simulink model "sim_battery_pack_simulink_with_EV_Load"  (R2021b)
settings: Solver=FixedStepAuto  StartTime=0.0  StopTime=3460.480  FixedStep=0.01  RelTol=1e-3
values from neighbouring files (symbols this model uses):
  Af = 1.4*1.6    (= 2.24)    [battery_pack_init_18_11.m]
  b = 0.002    [battery_pack_init_18_11.m]
  Batt_Eff = .98    (= 0.98)    [battery_pack_init_18_11.m]
  Batt_Ene_Cap = 7.37    [battery_pack_init_18_11.m]
  cd = 0.45    [battery_pack_init_18_11.m]
  dt = 0.01    [battery_pack_init_18_11.m]
  g = 9.81    [battery_pack_init_18_11.m]
  Gr = 5.75*.85    (= 4.8875)    [battery_pack_init_18_11.m]
  Grade = 7    [battery_pack_init_18_11.m]
  Ini_SOC = 100    [battery_pack_init_18_11.m]
  kappa = 0.1    [battery_pack_init_18_11.m]
  M = M_k+M_P    (= 445)    [battery_pack_init_18_11.m]
  M_Trq = T_m    [battery_pack_init_18_11.m]
  M_w = w_m    [battery_pack_init_18_11.m]
  Mot_Eff = .9    (= 0.9)    [battery_pack_init_18_11.m]
  mu = 0.016    [battery_pack_init_18_11.m]
  Np = 7    [battery_pack_init_18_11.m]
  Ns = 12    [battery_pack_init_18_11.m]
  Qgain = 1    [battery_pack_init_18_11.m]
  R0 = zeros(numpoles,1)    [battery_pack_init_18_11.m]
  R0Param = getParamESC('R0Param',T,cell_model)    [battery_pack_init_18_11.m]
  R_w = .3048/2    (= 0.1524)    [battery_pack_init_18_11.m]
  Re_spe_max = 50*5/18    (= 13.8888888889)    [battery_pack_init_18_11.m]
  Re_spe_min = 0*5/18    (= 0)    [battery_pack_init_18_11.m]
  rho = 1.225    [battery_pack_init_18_11.m]
  rt = .0008    (= 0.0008)    [battery_pack_init_18_11.m]
  T = 40    [battery_pack_init_18_11.m]
  T_MIDC = T_MIDC(1:72)    [battery_pack_init_18_11.m]
  Trans_Eff = .95    (= 0.95)    [battery_pack_init_18_11.m]
  V_MIDC = V_MIDC(1:72)    [battery_pack_init_18_11.m]
  Z0 = 0.75 + (1-0.75).*rand(1,Np)    [battery_pack_init_18_11.m]
undefined symbols (not defined in the file or in its folder): cell_model, FLbattery, gain, iload, sigbuilder_block, VMIDC
libraries: simulink x16, autolibshared x2, slpidlib x1, simulink_extras x1
(part 12 of 17)

== matlab function sim_battery_pack_simulink_with_EV_Load/SCM6/cell10/cell_model ==
  data: vk output size=1; T input; deltaT input; iR0 input; zkp input; irkp input; irkc output size=3; zkc output size=1; OCV output size=1; cell_model parameter; ik input; Qgain parameter

% function [vk,irk,hk,zk,sik,OCV] = simCell(ik,T,deltaT,model,z0,iR0,h0)
% 
% Simulates an ESC model for input current ik at temperature T
%
% Inputs:  ik - current, where (+) is discharge
%          T  - temperature (degC)
%      deltaT - sampling interval in data (s)
%       model - standard model structure
%          z0 - initial cell state of charge
%         iR0 - initial resistor currents as column vector
%          h0 - initial hysteresis state
% Outputs: vk - cell voltage for all timesteps
%         irk - resistor currents (in R-C branches) for all timesteps
%          hk - hysteresis states for all timesteps
%          zk - state of charge for all timesteps
%         sik - instantaneous hysteresis for all timesteps
%         OCV - open-circuit voltage for all timesteps

% Copyright (c) 2015 by Gregory L. Plett of the University of Colorado 
% Colorado Springs (UCCS). This work is licensed under a Creative Commons 
% Attribution-NonCommercial-ShareAlike 4.0 Intl. License, v. 1.0.
% It is provided "as is", without express or implied warranty, for 
% educational and informational purposes only.
%
% This file is provided as a supplement to: Plett, Gregory L., "Battery
% Management Systems, Volume I, Battery Modeling," Artech House, 2015.

function [vk,irkc,zkc,OCV] = cellmodel(T,deltaT,iR0, zkp,irkp, cell_model,ik, Qgain)
  % Force data to be column vector(s)
  
%   ik=[DYNData.script1.current(round(t*10)),DYNData.script1.current(round(t*10)+1)];
%   ik=interp1(0.1*(1:length(DYNData.script1.current)),DYNData.script1.current,t,'nearest');
  ik = ik(:); iR0 = iR0(:);
  
  % Get model parameters from model structure
  RCfact = exp(-deltaT./abs(getParamESC('RCParam',T,cell_model)))';
  Q = Qgain* getParamESC('QParam',T,cell_model);
  RParam = getParamESC('RParam',T,cell_model);
  R0Param = getParamESC('R0Param',T,cell_model);
  etaParam = getParamESC('etaParam',T,cell_model);
  
  etaik = ik; 
  for iii=1:length(ik)
    if etaik(iii)<0
        etaik(iii) = etaParam*ik(iii); % compensate for coulombic efficiency
    end
  end
  % Simulate the dynamic states of the model
  %if exist('ss','file'), % use control-system-toolbox method, if available
%     sysd= ss(diag(RCfact),1-RCfact,eye(length(RCfact)),0,0.1);
%     irk = lsim(sysd,etaik,[],iR0);
  %else
    irkc = RCfact.*irkp + (1-RCfact)*etaik(1);
  %end
%    irkc2 = irk(2,:)';
%    irkc=(irkc1+irkc2)/2;
  zkc = zkp-etaik(1)*deltaT/(Q*3600); 

    
  % Compute output equation
  OCV = OCVfromSOCtemp(zkc,T,cell_model);
  vk = OCV - RParam*irkc - ik(1).*R0Param ;%+ M*hk + M0*sik;
  
  


function theParam = getParamESC(paramName,temp,model)
%   theFields = fields(model); % get list of fields stored in model
%   match = strcmpi(paramName,theFields); % see if any match desired data
%   if ~match, % if not, throw an error
%     error('Parameter "%s" does not exist in model',paramName);
%   end
%   fieldName = char(theFields(match)); % case-sensitive field name

  % if model contains data at only one temperature
  if isscalar(model.temps),
    if model.temps ~= temp, % check whether requested data exists
      error('Model does not contain requested data at this temperature');
    end
    theParam = model.(paramName);
    return
  end

  % Otherwise, model has multiple temperatures. Bound input "temp" between
  % mininum and maximum stored temperature to prohibit "NaN" in output
  theParamData = model.(paramName);
  temp = max(min(temp,max(model.temps)),min(model.temps)); 
  ind = find(model.temps == temp); % see if there is an exact match to
  if ~isempty(ind), % avoid call to (slow) interp1 whenever possible
    if size(theParamData,1) == 1,
      theParam = theParamData(ind);
    else
      theParam = theParamData(ind,:);
    end
  else % if there is not an exact match, we interpolate between parameter
    theParam = interp1(model.temps,theParamData,temp,'spline'); % values
  end  % stored at different temperatures
  
  % function ocv = OCVfromSOCtemp(soc,temp,model)
%
% Computes the fully rested open-circuit voltage for a particular state of 
% charge and temperature point
%
% Inputs: soc = scalar or matrix of cell state of charge points
%        temp = scalar or matrix of temperatures at which to calc. OCV
%       model = data structure produced by processDynamic
% Output: ocv = scalar or matrix of open circuit voltages -- one for every
%               soc and temperature input point

% Copyright (c) 2015 by Gregory L. Plett of the University of Colorado 
% Colorado Springs (UCCS). This work is licensed under a Creative Commons 
% Attribution-NonCommercial-ShareAlike 4.0 Intl. License, v. 1.0.
% It is provided "as is", without express or implied warranty, for 
% educational and informational purposes only.
%
% This file is provided as a supplement to: Plett, Gregory L., "Battery
% Management Systems, Volume I, Battery Modeling," Artech House, 2015.

function ocv=OCVfromSOCtemp(soc,temp,model)
  soccol = soc(:); % force soc to be column vector
  SOC = model.SOC(:); % force to be column vector
  OCV0 = model.OCV0(:); % force to be column vector
  OCVrel = model.OCVrel(:); % force to be column vector
  if isscalar(temp), % replicate a scalar temperature for all socs
    tempcol = temp*ones(size(soccol)); 
  else
    tempcol = temp(:); % force matrix temperature to be column vector
    if ~isequal(size(tempcol),size(soccol)),
      error(['Function inputs "soc" and "temp" must either have same '...
        'number of elements, or "temp" must be a scalar']);
    end
  end
  diffSOC=SOC(2)-SOC(1); % spacing between SOC points - assume uniform
  ocv=zeros(size(soccol)); % initialize output to zero
  I1=find(soccol <= SOC(1)); % indices of socs below model-stored data
  I2=find(soccol >= SOC(end)); % and of socs above model-stored data
  I3=find(soccol > SOC(1) & soccol < SOC(end)); % the rest of them
  I6=isnan(soccol); % if input is "not a number" for any locations

  % for voltages less than lowest stored soc datapoint, extrapolate off 
  % low end of table 
  if ~isempty(I1),
    dv = (OCV0(2)+tempcol.*OCVrel(2)) - (OCV0(1)+tempcol.*OCVrel(1));
    ocv(I1)= (soccol(I1)-SOC(1)).*dv(I1)/diffSOC + ...
             OCV0(1)+tempcol(I1).*OCVrel(1);
  end

  % for voltages greater than highest stored soc datapoint, extrapolate off
  % high end of table
  if ~isempty(I2),
    dv = (OCV0(end)+tempcol.*OCVrel(end)) - ...
         (OCV0(end-1)+tempcol.*OCVrel(end-1));
    ocv(I2) = (soccol(I2)-SOC(end)).*dv(I2)/diffSOC + ...
              OCV0(end)+tempcol(I2).*OCVrel(end);
  end

  % for normal soc range, manually interpolate (10x faster than "interp1")
  I4=(soccol(I3)-SOC(1))/diffSOC; % using linear interpolation
  I5=floor(I4); I45 = I4-I5; omI45 = 1-I45;
  ocv(I3)=OCV0(I5+1).*omI45 + OCV0(I5+2).*I45;
  ocv(I3)=ocv(I3) + tempcol(I3).*(OCVrel(I5+1).*omI45 + OCVrel(I5+2).*I45);
  ocv(I6)=0; % replace NaN SOCs with zero voltage
  ocv = reshape(ocv,size(soc)); % output is same shape as input

== matlab function sim_battery_pack_simulink_with_EV_Load/SCM6/cell11/cell_model ==
  data: vk output size=1; T input; deltaT input; iR0 input; zkp input; irkp input; irkc output size=3; zkc output size=1; OCV output size=1; cell_model parameter; ik input; Qgain parameter

% function [vk,irk,hk,zk,sik,OCV] = simCell(ik,T,deltaT,model,z0,iR0,h0)
% 
% Simulates an ESC model for input current ik at temperature T
%
% Inputs:  ik - current, where (+) is discharge
%          T  - temperature (degC)
%      deltaT - sampling interval in data (s)
%       model - standard model structure
%          z0 - initial cell state of charge
%         iR0 - initial resistor currents as column vector
%          h0 - initial hysteresis state
% Outputs: vk - cell voltage for all timesteps
%         irk - resistor currents (in R-C branches) for all timesteps
%          hk - hysteresis states for all timesteps
%          zk - state of charge for all timesteps
%         sik - instantaneous hysteresis for all timesteps
%         OCV - open-circuit voltage for all timesteps

% Copyright (c) 2015 by Gregory L. Plett of the University of Colorado 
% Colorado Springs (UCCS). This work is licensed under a Creative Commons 
% Attribution-NonCommercial-ShareAlike 4.0 Intl. License, v. 1.0.
% It is provided "as is", without express or implied warranty, for 
% educational and informational purposes only.
%
% This file is provided as a supplement to: Plett, Gregory L., "Battery
% Management Systems, Volume I, Battery Modeling," Artech House, 2015.

function [vk,irkc,zkc,OCV] = cellmodel(T,deltaT,iR0, zkp,irkp, cell_model,ik, Qgain)
  % Force data to be column vector(s)
  
%   ik=[DYNData.script1.current(round(t*10)),DYNData.script1.current(round(t*10)+1)];
%   ik=interp1(0.1*(1:length(DYNData.script1.current)),DYNData.script1.current,t,'nearest');
  ik = ik(:); iR0 = iR0(:);
  
  % Get model parameters from model structure
  RCfact = exp(-deltaT./abs(getParamESC('RCParam',T,cell_model)))';
  Q = Qgain* getParamESC('QParam',T,cell_model);
  RParam = getParamESC('RParam',T,cell_model);
  R0Param = getParamESC('R0Param',T,cell_model);
  etaParam = getParamESC('etaParam',T,cell_model);
  
  etaik = ik; 
  for iii=1:length(ik)
    if etaik(iii)<0
        etaik(iii) = etaParam*ik(iii); % compensate for coulombic efficiency
    end
  end
  % Simulate the dynamic states of the model
  %if exist('ss','file'), % use control-system-toolbox method, if available
%     sysd= ss(diag(RCfact),1-RCfact,eye(length(RCfact)),0,0.1);
%     irk = lsim(sysd,etaik,[],iR0);
  %else
    irkc = RCfact.*irkp + (1-RCfact)*etaik(1);
  %end
%    irkc2 = irk(2,:)';
%    irkc=(irkc1+irkc2)/2;
  zkc = zkp-etaik(1)*deltaT/(Q*3600); 

    
  % Compute output equation
  OCV = OCVfromSOCtemp(zkc,T,cell_model);
  vk = OCV - RParam*irkc - ik(1).*R0Param ;%+ M*hk + M0*sik;
  
  


function theParam = getParamESC(paramName,temp,model)
%   theFields = fields(model); % get list of fields stored in model
%   match = strcmpi(paramName,theFields); % see if any match desired data
%   if ~match, % if not, throw an error
%     error('Parameter "%s" does not exist in model',paramName);
%   end
%   fieldName = char(theFields(match)); % case-sensitive field name

  % if model contains data at only one temperature
  if isscalar(model.temps),
    if model.temps ~= temp, % check whether requested data exists
      error('Model does not contain requested data at this temperature');
    end
    theParam = model.(paramName);
    return
  end

  % Otherwise, model has multiple temperatures. Bound input "temp" between
  % mininum and maximum stored temperature to prohibit "NaN" in output
  theParamData = model.(paramName);
  temp = max(min(temp,max(model.temps)),min(model.temps)); 
  ind = find(model.temps == temp); % see if there is an exact match to
  if ~isempty(ind), % avoid call to (slow) interp1 whenever possible
    if size(theParamData,1) == 1,
      theParam = theParamData(ind);
    else
      theParam = theParamData(ind,:);
    end
  else % if there is not an exact match, we interpolate between parameter
    theParam = interp1(model.temps,theParamData,temp,'spline'); % values
  end  % stored at different temperatures
  
  % function ocv = OCVfromSOCtemp(soc,temp,model)
%
% Computes the fully rested open-circuit voltage for a particular state of 
% charge and temperature point
%
% Inputs: soc = scalar or matrix of cell state of charge points
%        temp = scalar or matrix of temperatures at which to calc. OCV
%       model = data structure produced by processDynamic
% Output: ocv = scalar or matrix of open circuit voltages -- one for every
%               soc and temperature input point

% Copyright (c) 2015 by Gregory L. Plett of the University of Colorado 
% Colorado Springs (UCCS). This work is licensed under a Creative Commons 
% Attribution-NonCommercial-ShareAlike 4.0 Intl. License, v. 1.0.
% It is provided "as is", without express or implied warranty, for 
% educational and informational purposes only.
%
% This file is provided as a supplement to: Plett, Gregory L., "Battery
% Management Systems, Volume I, Battery Modeling," Artech House, 2015.

function ocv=OCVfromSOCtemp(soc,temp,model)
  soccol = soc(:); % force soc to be column vector
  SOC = model.SOC(:); % force to be column vector
  OCV0 = model.OCV0(:); % force to be column vector
  OCVrel = model.OCVrel(:); % force to be column vector
  if isscalar(temp), % replicate a scalar temperature for all socs
    tempcol = temp*ones(size(soccol)); 
  else
    tempcol = temp(:); % force matrix temperature to be column vector
    if ~isequal(size(tempcol),size(soccol)),
      error(['Function inputs "soc" and "temp" must either have same '...
        'number of elements, or "temp" must be a scalar']);
    end
  end
  diffSOC=SOC(2)-SOC(1); % spacing between SOC points - assume uniform
  ocv=zeros(size(soccol)); % initialize output to zero
  I1=find(soccol <= SOC(1)); % indices of socs below model-stored data
  I2=find(soccol >= SOC(end)); % and of socs above model-stored data
  I3=find(soccol > SOC(1) & soccol < SOC(end)); % the rest of them
  I6=isnan(soccol); % if input is "not a number" for any locations

  % for voltages less than lowest stored soc datapoint, extrapolate off 
  % low end of table 
  if ~isempty(I1),
    dv = (OCV0(2)+tempcol.*OCVrel(2)) - (OCV0(1)+tempcol.*OCVrel(1));
    ocv(I1)= (soccol(I1)-SOC(1)).*dv(I1)/diffSOC + ...
             OCV0(1)+tempcol(I1).*OCVrel(1);
  end

  % for voltages greater than highest stored soc datapoint, extrapolate off
  % high end of table
  if ~isempty(I2),
    dv = (OCV0(end)+tempcol.*OCVrel(end)) - ...
         (OCV0(end-1)+tempcol.*OCVrel(end-1));
    ocv(I2) = (soccol(I2)-SOC(end)).*dv(I2)/diffSOC + ...
              OCV0(end)+tempcol(I2).*OCVrel(end);
  end

  % for normal soc range, manually interpolate (10x faster than "interp1")
  I4=(soccol(I3)-SOC(1))/diffSOC; % using linear interpolation
  I5=floor(I4); I45 = I4-I5; omI45 = 1-I45;
  ocv(I3)=OCV0(I5+1).*omI45 + OCV0(I5+2).*I45;
  ocv(I3)=ocv(I3) + tempcol(I3).*(OCVrel(I5+1).*omI45 + OCVrel(I5+2).*I45);
  ocv(I6)=0; % replace NaN SOCs with zero voltage
  ocv = reshape(ocv,size(soc)); % output is same shape as input

== matlab function sim_battery_pack_simulink_with_EV_Load/SCM6/cell12/cell_model ==
  data: vk output size=1; T input; deltaT input; iR0 input; zkp input; irkp input; irkc output size=3; zkc output size=1; OCV output size=1; cell_model parameter; ik input; Qgain parameter

% function [vk,irk,hk,zk,sik,OCV] = simCell(ik,T,deltaT,model,z0,iR0,h0)
% 
% Simulates an ESC model for input current ik at temperature T
%
% Inputs:  ik - current, where (+) is discharge
%          T  - temperature (degC)
%      deltaT - sampling interval in data (s)
%       model - standard model structure
%          z0 - initial cell state of charge
%         iR0 - initial resistor currents as column vector
%          h0 - initial hysteresis state
% Outputs: vk - cell voltage for all timesteps
%         irk - resistor currents (in R-C branches) for all timesteps
%          hk - hysteresis states for all timesteps
%          zk - state of charge for all timesteps
%         sik - instantaneous hysteresis for all timesteps
%         OCV - open-circuit voltage for all timesteps

% Copyright (c) 2015 by Gregory L. Plett of the University of Colorado 
% Colorado Springs (UCCS). This work is licensed under a Creative Commons 
% Attribution-NonCommercial-ShareAlike 4.0 Intl. License, v. 1.0.
% It is provided "as is", without express or implied warranty, for 
% educational and informational purposes only.
%
% This file is provided as a supplement to: Plett, Gregory L., "Battery
% Management Systems, Volume I, Battery Modeling," Artech House, 2015.

function [vk,irkc,zkc,OCV] = cellmodel(T,deltaT,iR0, zkp,irkp, cell_model,ik, Qgain)
  % Force data to be column vector(s)
  
%   ik=[DYNData.script1.current(round(t*10)),DYNData.script1.current(round(t*10)+1)];
%   ik=interp1(0.1*(1:length(DYNData.script1.current)),DYNData.script1.current,t,'nearest');
  ik = ik(:); iR0 = iR0(:);
  
  % Get model parameters from model structure
  RCfact = exp(-deltaT./abs(getParamESC('RCParam',T,cell_model)))';
  Q = Qgain* getParamESC('QParam',T,cell_model);
  RParam = getParamESC('RParam',T,cell_model);
  R0Param = getParamESC('R0Param',T,cell_model);
  etaParam = getParamESC('etaParam',T,cell_model);
  
  etaik = ik; 
  for iii=1:length(ik)
    if etaik(iii)<0
        etaik(iii) = etaParam*ik(iii); % compensate for coulombic efficiency
    end
  end
  % Simulate the dynamic states of the model
  %if exist('ss','file'), % use control-system-toolbox method, if available
%     sysd= ss(diag(RCfact),1-RCfact,eye(length(RCfact)),0,0.1);
%     irk = lsim(sysd,etaik,[],iR0);
  %else
    irkc = RCfact.*irkp + (1-RCfact)*etaik(1);
  %end
%    irkc2 = irk(2,:)';
%    irkc=(irkc1+irkc2)/2;
  zkc = zkp-etaik(1)*deltaT/(Q*3600); 

    
  % Compute output equation
  OCV = OCVfromSOCtemp(zkc,T,cell_model);
  vk = OCV - RParam*irkc - ik(1).*R0Param ;%+ M*hk + M0*sik;
  
  


function theParam = getParamESC(paramName,temp,model)
%   theFields = fields(model); % get list of fields stored in model
%   match = strcmpi(paramName,theFields); % see if any match desired data
%   if ~match, % if not, throw an error
%     error('Parameter "%s" does not exist in model',paramName);
%   end
%   fieldName = char(theFields(match)); % case-sensitive field name

  % if model contains data at only one temperature
  if isscalar(model.temps),
    if model.temps ~= temp, % check whether requested data exists
      error('Model does not contain requested data at this temperature');
    end
    theParam = model.(paramName);
    return
  end

  % Otherwise, model has multiple temperatures. Bound input "temp" between
  % mininum and maximum stored temperature to prohibit "NaN" in output
  theParamData = model.(paramName);
  temp = max(min(temp,max(model.temps)),min(model.temps)); 
  ind = find(model.temps == temp); % see if there is an exact match to
  if ~isempty(ind), % avoid call to (slow) interp1 whenever possible
    if size(theParamData,1) == 1,
      theParam = theParamData(ind);
    else
      theParam = theParamData(ind,:);
    end
  else % if there is not an exact match, we interpolate between parameter
    theParam = interp1(model.temps,theParamData,temp,'spline'); % values
  end  % stored at different temperatures
  
  % function ocv = OCVfromSOCtemp(soc,temp,model)
%
% Computes the fully rested open-circuit voltage for a particular state of 
% charge and temperature point
%
% Inputs: soc = scalar or matrix of cell state of charge points
%        temp = scalar or matrix of temperatures at which to calc. OCV
%       model = data structure produced by processDynamic
% Output: ocv = scalar or matrix of open circuit voltages -- one for every
%               soc and temperature input point

% Copyright (c) 2015 by Gregory L. Plett of the University of Colorado 
% Colorado Springs (UCCS). This work is licensed under a Creative Commons 
% Attribution-NonCommercial-ShareAlike 4.0 Intl. License, v. 1.0.
% It is provided "as is", without express or implied warranty, for 
% educational and informational purposes only.
%
% This file is provided as a supplement to: Plett, Gregory L., "Battery
% Management Systems, Volume I, Battery Modeling," Artech House, 2015.

function ocv=OCVfromSOCtemp(soc,temp,model)
  soccol = soc(:); % force soc to be column vector
  SOC = model.SOC(:); % force to be column vector
  OCV0 = model.OCV0(:); % force to be column vector
  OCVrel = model.OCVrel(:); % force to be column vector
  if isscalar(temp), % replicate a scalar temperature for all socs
    tempcol = temp*ones(size(soccol)); 
  else
    tempcol = temp(:); % force matrix temperature to be column vector
    if ~isequal(size(tempcol),size(soccol)),
      error(['Function inputs "soc" and "temp" must either have same '...
        'number of elements, or "temp" must be a scalar']);
    end
  end
  diffSOC=SOC(2)-SOC(1); % spacing between SOC points - assume uniform
  ocv=zeros(size(soccol)); % initialize output to zero
  I1=find(soccol <= SOC(1)); % indices of socs below model-stored data
  I2=find(soccol >= SOC(end)); % and of socs above model-stored data
  I3=find(soccol > SOC(1) & soccol < SOC(end)); % the rest of them
  I6=isnan(soccol); % if input is "not a number" for any locations

  % for voltages less than lowest stored soc datapoint, extrapolate off 
  % low end of table 
  if ~isempty(I1),
    dv = (OCV0(2)+tempcol.*OCVrel(2)) - (OCV0(1)+tempcol.*OCVrel(1));
    ocv(I1)= (soccol(I1)-SOC(1)).*dv(I1)/diffSOC + ...
             OCV0(1)+tempcol(I1).*OCVrel(1);
  end

  % for voltages greater than highest stored soc datapoint, extrapolate off
  % high end of table
  if ~isempty(I2),
    dv = (OCV0(end)+tempcol.*OCVrel(end)) - ...
         (OCV0(end-1)+tempcol.*OCVrel(end-1));
    ocv(I2) = (soccol(I2)-SOC(end)).*dv(I2)/diffSOC + ...
              OCV0(end)+tempcol(I2).*OCVrel(end);
  end

  % for normal soc range, manually interpolate (10x faster than "interp1")
  I4=(soccol(I3)-SOC(1))/diffSOC; % using linear interpolation
  I5=floor(I4); I45 = I4-I5; omI45 = 1-I45;
  ocv(I3)=OCV0(I5+1).*omI45 + OCV0(I5+2).*I45;
  ocv(I3)=ocv(I3) + tempcol(I3).*(OCVrel(I5+1).*omI45 + OCVrel(I5+2).*I45);
  ocv(I6)=0; % replace NaN SOCs with zero voltage
  ocv = reshape(ocv,size(soc)); % output is same shape as input

== matlab function sim_battery_pack_simulink_with_EV_Load/SCM6/cell2/cell_model ==
  data: vk output size=1; T input; deltaT input; iR0 input; zkp input; irkp input; irkc output size=3; zkc output size=1; OCV output size=1; cell_model parameter; ik input; Qgain parameter

% function [vk,irk,hk,zk,sik,OCV] = simCell(ik,T,deltaT,model,z0,iR0,h0)
% 
% Simulates an ESC model for input current ik at temperature T
%
% Inputs:  ik - current, where (+) is discharge
%          T  - temperature (degC)
%      deltaT - sampling interval in data (s)
%       model - standard model structure
%          z0 - initial cell state of charge
%         iR0 - initial resistor currents as column vector
%          h0 - initial hysteresis state
% Outputs: vk - cell voltage for all timesteps
%         irk - resistor currents (in R-C branches) for all timesteps
%          hk - hysteresis states for all timesteps
%          zk - state of charge for all timesteps
%         sik - instantaneous hysteresis for all timesteps
%         OCV - open-circuit voltage for all timesteps

% Copyright (c) 2015 by Gregory L. Plett of the University of Colorado 
% Colorado Springs (UCCS). This work is licensed under a Creative Commons 
% Attribution-NonCommercial-ShareAlike 4.0 Intl. License, v. 1.0.
% It is provided "as is", without express or implied warranty, for 
% educational and informational purposes only.
%
% This file is provided as a supplement to: Plett, Gregory L., "Battery
% Management Systems, Volume I, Battery Modeling," Artech House, 2015.

function [vk,irkc,zkc,OCV] = cellmodel(T,deltaT,iR0, zkp,irkp, cell_model,ik, Qgain)
  % Force data to be column vector(s)
  
%   ik=[DYNData.script1.current(round(t*10)),DYNData.script1.current(round(t*10)+1)];
%   ik=interp1(0.1*(1:length(DYNData.script1.current)),DYNData.script1.current,t,'nearest');
  ik = ik(:); iR0 = iR0(:);
  
  % Get model parameters from model structure
  RCfact = exp(-deltaT./abs(getParamESC('RCParam',T,cell_model)))';
  Q = Qgain* getParamESC('QParam',T,cell_model);
  RParam = getParamESC('RParam',T,cell_model);
  R0Param = getParamESC('R0Param',T,cell_model);
  etaParam = getParamESC('etaParam',T,cell_model);
  
  etaik = ik; 
  for iii=1:length(ik)
    if etaik(iii)<0
        etaik(iii) = etaParam*ik(iii); % compensate for coulombic efficiency
    end
  end
  % Simulate the dynamic states of the model
  %if exist('ss','file'), % use control-system-toolbox method, if available
%     sysd= ss(diag(RCfact),1-RCfact,eye(length(RCfact)),0,0.1);
%     irk = lsim(sysd,etaik,[],iR0);
  %else
    irkc = RCfact.*irkp + (1-RCfact)*etaik(1);
  %end
%    irkc2 = irk(2,:)';
%    irkc=(irkc1+irkc2)/2;
  zkc = zkp-etaik(1)*deltaT/(Q*3600); 

    
  % Compute output equation
  OCV = OCVfromSOCtemp(zkc,T,cell_model);
  vk = OCV - RParam*irkc - ik(1).*R0Param ;%+ M*hk + M0*sik;
  
  


function theParam = getParamESC(paramName,temp,model)
%   theFields = fields(model); % get list of fields stored in model
%   match = strcmpi(paramName,theFields); % see if any match desired data
%   if ~match, % if not, throw an error
%     error('Parameter "%s" does not exist in model',paramName);
%   end
%   fieldName = char(theFields(match)); % case-sensitive field name

  % if model contains data at only one temperature
  if isscalar(model.temps),
    if model.temps ~= temp, % check whether requested data exists
      error('Model does not contain requested data at this temperature');
    end
    theParam = model.(paramName);
    return
  end

  % Otherwise, model has multiple temperatures. Bound input "temp" between
  % mininum and maximum stored temperature to prohibit "NaN" in output
  theParamData = model.(paramName);
  temp = max(min(temp,max(model.temps)),min(model.temps)); 
  ind = find(model.temps == temp); % see if there is an exact match to
  if ~isempty(ind), % avoid call to (slow) interp1 whenever possible
    if size(theParamData,1) == 1,
      theParam = theParamData(ind);
    else
      theParam = theParamData(ind,:);
    end
  else % if there is not an exact match, we interpolate between parameter
    theParam = interp1(model.temps,theParamData,temp,'spline'); % values
  end  % stored at different temperatures
  
  % function ocv = OCVfromSOCtemp(soc,temp,model)
%
% Computes the fully rested open-circuit voltage for a particular state of 
% charge and temperature point
%
% Inputs: soc = scalar or matrix of cell state of charge points
%        temp = scalar or matrix of temperatures at which to calc. OCV
%       model = data structure produced by processDynamic
% Output: ocv = scalar or matrix of open circuit voltages -- one for every
%               soc and temperature input point

% Copyright (c) 2015 by Gregory L. Plett of the University of Colorado 
% Colorado Springs (UCCS). This work is licensed under a Creative Commons 
% Attribution-NonCommercial-ShareAlike 4.0 Intl. License, v. 1.0.
% It is provided "as is", without express or implied warranty, for 
% educational and informational purposes only.
%
% This file is provided as a supplement to: Plett, Gregory L., "Battery
% Management Systems, Volume I, Battery Modeling," Artech House, 2015.

function ocv=OCVfromSOCtemp(soc,temp,model)
  soccol = soc(:); % force soc to be column vector
  SOC = model.SOC(:); % force to be column vector
  OCV0 = model.OCV0(:); % force to be column vector
  OCVrel = model.OCVrel(:); % force to be column vector
  if isscalar(temp), % replicate a scalar temperature for all socs
    tempcol = temp*ones(size(soccol)); 
  else
    tempcol = temp(:); % force matrix temperature to be column vector
    if ~isequal(size(tempcol),size(soccol)),
      error(['Function inputs "soc" and "temp" must either have same '...
        'number of elements, or "temp" must be a scalar']);
    end
  end
  diffSOC=SOC(2)-SOC(1); % spacing between SOC points - assume uniform
  ocv=zeros(size(soccol)); % initialize output to zero
  I1=find(soccol <= SOC(1)); % indices of socs below model-stored data
  I2=find(soccol >= SOC(end)); % and of socs above model-stored data
  I3=find(soccol > SOC(1) & soccol < SOC(end)); % the rest of them
  I6=isnan(soccol); % if input is "not a number" for any locations

  % for voltages less than lowest stored soc datapoint, extrapolate off 
  % low end of table 
  if ~isempty(I1),
    dv = (OCV0(2)+tempcol.*OCVrel(2)) - (OCV0(1)+tempcol.*OCVrel(1));
    ocv(I1)= (soccol(I1)-SOC(1)).*dv(I1)/diffSOC + ...
             OCV0(1)+tempcol(I1).*OCVrel(1);
  end

  % for voltages greater than highest stored soc datapoint, extrapolate off
  % high end of table
  if ~isempty(I2),
    dv = (OCV0(end)+tempcol.*OCVrel(end)) - ...
         (OCV0(end-1)+tempcol.*OCVrel(end-1));
    ocv(I2) = (soccol(I2)-SOC(end)).*dv(I2)/diffSOC + ...
              OCV0(end)+tempcol(I2).*OCVrel(end);
  end

  % for normal soc range, manually interpolate (10x faster than "interp1")
  I4=(soccol(I3)-SOC(1))/diffSOC; % using linear interpolation
  I5=floor(I4); I45 = I4-I5; omI45 = 1-I45;
  ocv(I3)=OCV0(I5+1).*omI45 + OCV0(I5+2).*I45;
  ocv(I3)=ocv(I3) + tempcol(I3).*(OCVrel(I5+1).*omI45 + OCVrel(I5+2).*I45);
  ocv(I6)=0; % replace NaN SOCs with zero voltage
  ocv = reshape(ocv,size(soc)); % output is same shape as input

== matlab function sim_battery_pack_simulink_with_EV_Load/SCM6/cell3/cell_model ==
  data: vk output size=1; T input; deltaT input; iR0 input; zkp input; irkp input; irkc output size=3; zkc output size=1; OCV output size=1; cell_model parameter; ik input; Qgain parameter

% function [vk,irk,hk,zk,sik,OCV] = simCell(ik,T,deltaT,model,z0,iR0,h0)
% 
% Simulates an ESC model for input current ik at temperature T
%
% Inputs:  ik - current, where (+) is discharge
%          T  - temperature (degC)
%      deltaT - sampling interval in data (s)
%       model - standard model structure
%          z0 - initial cell state of charge
%         iR0 - initial resistor currents as column vector
%          h0 - initial hysteresis state
% Outputs: vk - cell voltage for all timesteps
%         irk - resistor currents (in R-C branches) for all timesteps
%          hk - hysteresis states for all timesteps
%          zk - state of charge for all timesteps
%         sik - instantaneous hysteresis for all timesteps
%         OCV - open-circuit voltage for all timesteps

% Copyright (c) 2015 by Gregory L. Plett of the University of Colorado 
% Colorado Springs (UCCS). This work is licensed under a Creative Commons 
% Attribution-NonCommercial-ShareAlike 4.0 Intl. License, v. 1.0.
% It is provided "as is", without express or implied warranty, for 
% educational and informational purposes only.
%
% This file is provided as a supplement to: Plett, Gregory L., "Battery
% Management Systems, Volume I, Battery Modeling," Artech House, 2015.

function [vk,irkc,zkc,OCV] = cellmodel(T,deltaT,iR0, zkp,irkp, cell_model,ik, Qgain)
  % Force data to be column vector(s)
  
%   ik=[DYNData.script1.current(round(t*10)),DYNData.script1.current(round(t*10)+1)];
%   ik=interp1(0.1*(1:length(DYNData.script1.current)),DYNData.script1.current,t,'nearest');
  ik = ik(:); iR0 = iR0(:);
  
  % Get model parameters from model structure
  RCfact = exp(-deltaT./abs(getParamESC('RCParam',T,cell_model)))';
  Q = Qgain* getParamESC('QParam',T,cell_model);
  RParam = getParamESC('RParam',T,cell_model);
  R0Param = getParamESC('R0Param',T,cell_model);
  etaParam = getParamESC('etaParam',T,cell_model);
  
  etaik = ik; 
  for iii=1:length(ik)
    if etaik(iii)<0
        etaik(iii) = etaParam*ik(iii); % compensate for coulombic efficiency
    end
  end
  % Simulate the dynamic states of the model
  %if exist('ss','file'), % use control-system-toolbox method, if available
%     sysd= ss(diag(RCfact),1-RCfact,eye(length(RCfact)),0,0.1);
%     irk = lsim(sysd,etaik,[],iR0);
  %else
    irkc = RCfact.*irkp + (1-RCfact)*etaik(1);
  %end
%    irkc2 = irk(2,:)';
%    irkc=(irkc1+irkc2)/2;
  zkc = zkp-etaik(1)*deltaT/(Q*3600); 

    
  % Compute output equation
  OCV = OCVfromSOCtemp(zkc,T,cell_model);
  vk = OCV - RParam*irkc - ik(1).*R0Param ;%+ M*hk + M0*sik;
  
  


function theParam = getParamESC(paramName,temp,model)
%   theFields = fields(model); % get list of fields stored in model
%   match = strcmpi(paramName,theFields); % see if any match desired data
%   if ~match, % if not, throw an error
%     error('Parameter "%s" does not exist in model',paramName);
%   end
%   fieldName = char(theFields(match)); % case-sensitive field name

  % if model contains data at only one temperature
  if isscalar(model.temps),
    if model.temps ~= temp, % check whether requested data exists
      error('Model does not contain requested data at this temperature');
    end
    theParam = model.(paramName);
    return
  end

  % Otherwise, model has multiple temperatures. Bound input "temp" between
  % mininum and maximum stored temperature to prohibit "NaN" in output
  theParamData = model.(paramName);
  temp = max(min(temp,max(model.temps)),min(model.temps)); 
  ind = find(model.temps == temp); % see if there is an exact match to
  if ~isempty(ind), % avoid call to (slow) interp1 whenever possible
    if size(theParamData,1) == 1,
      theParam = theParamData(ind);
    else
      theParam = theParamData(ind,:);
    end
  else % if there is not an exact match, we interpolate between parameter
    theParam = interp1(model.temps,theParamData,temp,'spline'); % values
  end  % stored at different temperatures
  
  % function ocv = OCVfromSOCtemp(soc,temp,model)
%
% Computes the fully rested open-circuit voltage for a particular state of 
% charge and temperature point
%
% Inputs: soc = scalar or matrix of cell state of charge points
%        temp = scalar or matrix of temperatures at which to calc. OCV
%       model = data structure produced by processDynamic
% Output: ocv = scalar or matrix of open circuit voltages -- one for every
%               soc and temperature input point

% Copyright (c) 2015 by Gregory L. Plett of the University of Colorado 
% Colorado Springs (UCCS). This work is licensed under a Creative Commons 
% Attribution-NonCommercial-ShareAlike 4.0 Intl. License, v. 1.0.
% It is provided "as is", without express or implied warranty, for 
% educational and informational purposes only.
%
% This file is provided as a supplement to: Plett, Gregory L., "Battery
% Management Systems, Volume I, Battery Modeling," Artech House, 2015.

function ocv=OCVfromSOCtemp(soc,temp,model)
  soccol = soc(:); % force soc to be column vector
  SOC = model.SOC(:); % force to be column vector
  OCV0 = model.OCV0(:); % force to be column vector
  OCVrel = model.OCVrel(:); % force to be column vector
  if isscalar(temp), % replicate a scalar temperature for all socs
    tempcol = temp*ones(size(soccol)); 
  else
    tempcol = temp(:); % force matrix temperature to be column vector
    if ~isequal(size(tempcol),size(soccol)),
      error(['Function inputs "soc" and "temp" must either have same '...
        'number of elements, or "temp" must be a scalar']);
    end
  end
  diffSOC=SOC(2)-SOC(1); % spacing between SOC points - assume uniform
  ocv=zeros(size(soccol)); % initialize output to zero
  I1=find(soccol <= SOC(1)); % indices of socs below model-stored data
  I2=find(soccol >= SOC(end)); % and of socs above model-stored data
  I3=find(soccol > SOC(1) & soccol < SOC(end)); % the rest of them
  I6=isnan(soccol); % if input is "not a number" for any locations

  % for voltages less than lowest stored soc datapoint, extrapolate off 
  % low end of table 
  if ~isempty(I1),
    dv = (OCV0(2)+tempcol.*OCVrel(2)) - (OCV0(1)+tempcol.*OCVrel(1));
    ocv(I1)= (soccol(I1)-SOC(1)).*dv(I1)/diffSOC + ...
             OCV0(1)+tempcol(I1).*OCVrel(1);
  end

  % for voltages greater than highest stored soc datapoint, extrapolate off
  % high end of table
  if ~isempty(I2),
    dv = (OCV0(end)+tempcol.*OCVrel(end)) - ...
         (OCV0(end-1)+tempcol.*OCVrel(end-1));
    ocv(I2) = (soccol(I2)-SOC(end)).*dv(I2)/diffSOC + ...
              OCV0(end)+tempcol(I2).*OCVrel(end);
  end

  % for normal soc range, manually interpolate (10x faster than "interp1")
  I4=(soccol(I3)-SOC(1))/diffSOC; % using linear interpolation
  I5=floor(I4); I45 = I4-I5; omI45 = 1-I45;
  ocv(I3)=OCV0(I5+1).*omI45 + OCV0(I5+2).*I45;
  ocv(I3)=ocv(I3) + tempcol(I3).*(OCVrel(I5+1).*omI45 + OCVrel(I5+2).*I45);
  ocv(I6)=0; % replace NaN SOCs with zero voltage
  ocv = reshape(ocv,size(soc)); % output is same shape as input

== matlab function sim_battery_pack_simulink_with_EV_Load/SCM6/cell4/cell_model ==
  data: vk output size=1; T input; deltaT input; iR0 input; zkp input; irkp input; irkc output size=3; zkc output size=1; OCV output size=1; cell_model parameter; ik input; Qgain parameter

% function [vk,irk,hk,zk,sik,OCV] = simCell(ik,T,deltaT,model,z0,iR0,h0)
% 
% Simulates an ESC model for input current ik at temperature T
%
% Inputs:  ik - current, where (+) is discharge
%          T  - temperature (degC)
%      deltaT - sampling interval in data (s)
%       model - standard model structure
%          z0 - initial cell state of charge
%         iR0 - initial resistor currents as column vector
%          h0 - initial hysteresis state
% Outputs: vk - cell voltage for all timesteps
%         irk - resistor currents (in R-C branches) for all timesteps
%          hk - hysteresis states for all timesteps
%          zk - state of charge for all timesteps
%         sik - instantaneous hysteresis for all timesteps
%         OCV - open-circuit voltage for all timesteps

% Copyright (c) 2015 by Gregory L. Plett of the University of Colorado 
% Colorado Springs (UCCS). This work is licensed under a Creative Commons 
% Attribution-NonCommercial-ShareAlike 4.0 Intl. License, v. 1.0.
% It is provided "as is", without express or implied warranty, for 
% educational and informational purposes only.
%
% This file is provided as a supplement to: Plett, Gregory L., "Battery
% Management Systems, Volume I, Battery Modeling," Artech House, 2015.

function [vk,irkc,zkc,OCV] = cellmodel(T,deltaT,iR0, zkp,irkp, cell_model,ik, Qgain)
  % Force data to be column vector(s)
  
%   ik=[DYNData.script1.current(round(t*10)),DYNData.script1.current(round(t*10)+1)];
%   ik=interp1(0.1*(1:length(DYNData.script1.current)),DYNData.script1.current,t,'nearest');
  ik = ik(:); iR0 = iR0(:);
  
  % Get model parameters from model structure
  RCfact = exp(-deltaT./abs(getParamESC('RCParam',T,cell_model)))';
  Q = Qgain* getParamESC('QParam',T,cell_model);
  RParam = getParamESC('RParam',T,cell_model);
  R0Param = getParamESC('R0Param',T,cell_model);
  etaParam = getParamESC('etaParam',T,cell_model);
  
  etaik = ik; 
  for iii=1:length(ik)
    if etaik(iii)<0
        etaik(iii) = etaParam*ik(iii); % compensate for coulombic efficiency
    end
  end
  % Simulate the dynamic states of the model
  %if exist('ss','file'), % use control-system-toolbox method, if available
%     sysd= ss(diag(RCfact),1-RCfact,eye(length(RCfact)),0,0.1);
%     irk = lsim(sysd,etaik,[],iR0);
  %else
    irkc = RCfact.*irkp + (1-RCfact)*etaik(1);
  %end
%    irkc2 = irk(2,:)';
%    irkc=(irkc1+irkc2)/2;
  zkc = zkp-etaik(1)*deltaT/(Q*3600); 

    
  % Compute output equation
  OCV = OCVfromSOCtemp(zkc,T,cell_model);
  vk = OCV - RParam*irkc - ik(1).*R0Param ;%+ M*hk + M0*sik;
  
  


function theParam = getParamESC(paramName,temp,model)
%   theFields = fields(model); % get list of fields stored in model
%   match = strcmpi(paramName,theFields); % see if any match desired data
%   if ~match, % if not, throw an error
%     error('Parameter "%s" does not exist in model',paramName);
%   end
%   fieldName = char(theFields(match)); % case-sensitive field name

  % if model contains data at only one temperature
  if isscalar(model.temps),
    if model.temps ~= temp, % check whether requested data exists
      error('Model does not contain requested data at this temperature');
    end
    theParam = model.(paramName);
    return
  end

  % Otherwise, model has multiple temperatures. Bound input "temp" between
  % mininum and maximum stored temperature to prohibit "NaN" in output
  theParamData = model.(paramName);
  temp = max(min(temp,max(model.temps)),min(model.temps)); 
  ind = find(model.temps == temp); % see if there is an exact match to
  if ~isempty(ind), % avoid call to (slow) interp1 whenever possible
    if size(theParamData,1) == 1,
      theParam = theParamData(ind);
    else
      theParam = theParamData(ind,:);
    end
  else % if there is not an exact match, we interpolate between parameter
    theParam = interp1(model.temps,theParamData,temp,'spline'); % values
  end  % stored at different temperatures
  
  % function ocv = OCVfromSOCtemp(soc,temp,model)
%
% Computes the fully rested open-circuit voltage for a particular state of 
% charge and temperature point
%
% Inputs: soc = scalar or matrix of cell state of charge points
%        temp = scalar or matrix of temperatures at which to calc. OCV
%       model = data structure produced by processDynamic
% Output: ocv = scalar or matrix of open circuit voltages -- one for every
%               soc and temperature input point

% Copyright (c) 2015 by Gregory L. Plett of the University of Colorado 
% Colorado Springs (UCCS). This work is licensed under a Creative Commons 
% Attribution-NonCommercial-ShareAlike 4.0 Intl. License, v. 1.0.
% It is provided "as is", without express or implied warranty, for 
% educational and informational purposes only.
%
% This file is provided as a supplement to: Plett, Gregory L., "Battery
% Management Systems, Volume I, Battery Modeling," Artech House, 2015.

function ocv=OCVfromSOCtemp(soc,temp,model)
  soccol = soc(:); % force soc to be column vector
  SOC = model.SOC(:); % force to be column vector
  OCV0 = model.OCV0(:); % force to be column vector
  OCVrel = model.OCVrel(:); % force to be column vector
  if isscalar(temp), % replicate a scalar temperature for all socs
    tempcol = temp*ones(size(soccol)); 
  else
    tempcol = temp(:); % force matrix temperature to be column vector
    if ~isequal(size(tempcol),size(soccol)),
      error(['Function inputs "soc" and "temp" must either have same '...
        'number of elements, or "temp" must be a scalar']);
    end
  end
  diffSOC=SOC(2)-SOC(1); % spacing between SOC points - assume uniform
  ocv=zeros(size(soccol)); % initialize output to zero
  I1=find(soccol <= SOC(1)); % indices of socs below model-stored data
  I2=find(soccol >= SOC(end)); % and of socs above model-stored data
  I3=find(soccol > SOC(1) & soccol < SOC(end)); % the rest of them
  I6=isnan(soccol); % if input is "not a number" for any locations

  % for voltages less than lowest stored soc datapoint, extrapolate off 
  % low end of table 
  if ~isempty(I1),
    dv = (OCV0(2)+tempcol.*OCVrel(2)) - (OCV0(1)+tempcol.*OCVrel(1));
    ocv(I1)= (soccol(I1)-SOC(1)).*dv(I1)/diffSOC + ...
             OCV0(1)+tempcol(I1).*OCVrel(1);
  end

  % for voltages greater than highest stored soc datapoint, extrapolate off
  % high end of table
  if ~isempty(I2),
    dv = (OCV0(end)+tempcol.*OCVrel(end)) - ...
         (OCV0(end-1)+tempcol.*OCVrel(end-1));
    ocv(I2) = (soccol(I2)-SOC(end)).*dv(I2)/diffSOC + ...
              OCV0(end)+tempcol(I2).*OCVrel(end);
  end

  % for normal soc range, manually interpolate (10x faster than "interp1")
  I4=(soccol(I3)-SOC(1))/diffSOC; % using linear interpolation
  I5=floor(I4); I45 = I4-I5; omI45 = 1-I45;
  ocv(I3)=OCV0(I5+1).*omI45 + OCV0(I5+2).*I45;
  ocv(I3)=ocv(I3) + tempcol(I3).*(OCVrel(I5+1).*omI45 + OCVrel(I5+2).*I45);
  ocv(I6)=0; % replace NaN SOCs with zero voltage
  ocv = reshape(ocv,size(soc)); % output is same shape as input
